simulink model "Diff_UG_2020a"  (R2020a)
settings: Solver=ode3  StartTime=0.0  StopTime=0.2  FixedStep=1e-6  RelTol=1e-3
InitFcn:
  | Ts=1/1200;
StartFcn:
  | Ts=1/1200;
undefined symbols (not defined in the file): powergui, spspowerguiLib
libraries: simulink x5, spsFourierLib x5, spsThreePhaseVIMeasurementLib x4, spsDistributedParametersLineLib x2, spsThreePhaseFaultLib x1, spsThreePhaseSeriesRLCLoadLib x1, spsThreePhaseTransformerTwoWindingsLib x1, spsThreePhaseBreakerLib x1, spsThreePhaseSourceLib x1
settings Model: Creator=AMLAN SWAIN  LastModifiedBy=mluser
settings SolverCC: ZeroCrossAlgorithm=Adaptive
settings DataIOCC: SaveFormat=StructureWithTime  ReturnWorkspaceOutputs=off
settings OptimizationCC: LifeSpan=inf
settings DebuggingCC: IgnoredZcDiagnostic=none  FcnCallInpInsideContextMsg=warning  SFExecutionAtInitializationDiag=none  ArithmeticOperatorsInVariantConditions=warning
settings HardwareCC: ProdBitPerSizeT=32  ProdBitPerPtrDiffT=32  ProdWordSize=32  ProdHWDeviceType=Specified
settings SFSimCC: CustomCodeUndefinedFunction=UseInterfaceOnly
settings CodeAppCC: StateflowObjectComments=on

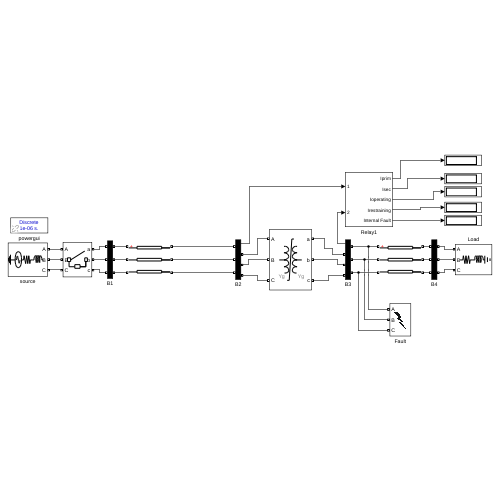
[thumbnail: Simulink's stored preview of the top-level diagram]
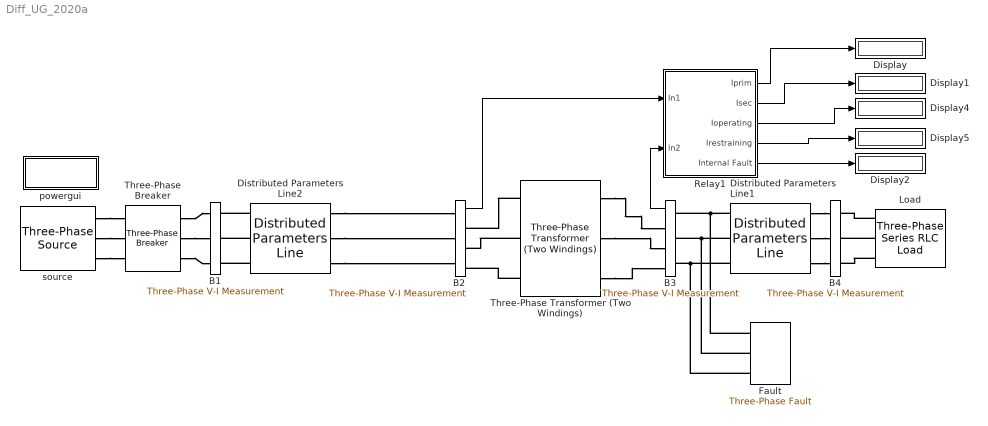
== system Diff_UG_2020a ==
  B1 : spsThreePhaseVIMeasurementLib/Three-Phase V-I Measurement  VoltageMeasurement=phase-to-phase  SetLabelV=on  LabelV=Vabc_B1  Vpu=off  VpuLL=off  CurrentMeasurement=yes  SetLabelI=on  LabelI=Iabc_B1  Ipu=off  Pbase=100e6  Vbase=500e3  OutputType=Complex  PhasorSimulation=off  PSBequivalent=0
  B2 : spsThreePhaseVIMeasurementLib/Three-Phase V-I Measurement  VoltageMeasurement=phase-to-phase  SetLabelV=on  LabelV=Vabc_B2  Vpu=off  VpuLL=off  CurrentMeasurement=yes  SetLabelI=off  LabelI=Iabc_B2  Ipu=off  Pbase=100e6  Vbase=500e3  OutputType=Complex  PhasorSimulation=off  PSBequivalent=0
  B3 : spsThreePhaseVIMeasurementLib/Three-Phase V-I Measurement  VoltageMeasurement=phase-to-phase  SetLabelV=on  LabelV=Vabc_B3  Vpu=off  VpuLL=off  CurrentMeasurement=yes  SetLabelI=off  LabelI=Iabc_B3  Ipu=off  Pbase=100e6  Vbase=500e3  OutputType=Complex  PhasorSimulation=off  PSBequivalent=0
  B4 : spsThreePhaseVIMeasurementLib/Three-Phase V-I Measurement  VoltageMeasurement=phase-to-phase  SetLabelV=on  LabelV=Vabc_B4  Vpu=off  VpuLL=off  CurrentMeasurement=yes  SetLabelI=on  LabelI=Iabc_B5  Ipu=off  Pbase=100e6  Vbase=500e3  OutputType=Complex  PhasorSimulation=off  PSBequivalent=0
  Display{,1..2,4..5} (5 alike) : Display
  Distributed Parameters Line1 : spsDistributedParametersLineLib/Distributed Parameters Line  Phases=3  Length=0.762  Frequency=60  Resistance=[0.306 0.5919]/1.6  Inductance="[0.6272  2.9855]/(2*3.14*60*1.6)"  Capacitance=[12.74e-9 7.751e-9]  x1=[-5e-06 1.09405688634751e-10 72.6531448887582 -51.7681554973917;-4e-06 1.09439141081101e-10 72.6726558603192 -51.7407622289867;-3e-06 1.09472577973709e-10 72.6921565034752 -51.7133616070655;-2e-06 1.09505999307821e-10 72.7116468154545 -51.6859536355223;-1e-06 1.09539405078689e-10 72.7311267934873 -51.6585383182524]  x2=[-5e-06 1.00008983678e-10 71.2021479909671 -51.8216475042181;-4e-06 1.00043099451765e-10 71.2216792316487 -51.7948012449423;-3e-06 1.00077201007175e-10 71.2412003501413 -51.7679476244701;-2e-06 1.00111288339383e-10 71.2607113436705 -51.741086646618;-1e-06 1.00145361443545e-10 71.2802122094634 -51.7142183152036]  x3=[-5e-06 -2.29756752635099e-12 -1.80275880533719 3.66974532044683;-4e-06 -2.29982601994123e-12 -1.80414213859099 3.66906543562833;-3e-06 -2.30208418667492e-12 -1.80552521543596 3.66838502935381;-2e-06 -2.30434202623109e-12 -1.80690803567553 3.66770410171997;-1e-06 -2.30659953828888e-12 -1.80829059911317 3.66702265282357]  x4=[-5e-06 2.59243524442771e-12 2.305788104249 -4.03237498109375;-4e-06 2.59477372905035e-12 2.30730810991507 -4.03150543293286;-3e-06 2.59711184489777e-12 2.30882778766119 -4.03063531180515;-2e-06 2.59944959163768e-12 2.31034713727139 -4.02976461783426;-1e-06 2.60178696893783e-12 2.31186615852974 -4.02889335114395]  x5=4.72092324098614e-06  V1=[9.374e-10 1.076e+04 1.076e+04;377 377 377;-1.988 0.4876 -1.083]  V2=[8.927e-10 1.062e+04 1.062e+04;377 377 377;-2.049 0.4776 -1.093]  I1=[5.305e-11 493.3 493.3;377 377 377;0.5859 3.134 1.563]  I2=[5.319e-11 560.4 560.4;377 377 377;-2.484 0.05536 -1.515]  nHarmo=1  Measurements=None  Decoupling=off  VsMag0=0  VrMag0=0  VsAngle0=0  VrAngle0=0  IsMag0=0  IrMag0=0  IsAngle0=0  IrAngle0=0
      settings: SourceProductBaseCode=PS
  Distributed Parameters Line2 : spsDistributedParametersLineLib/Distributed Parameters Line  Phases=3  Length=0.609  Frequency=60  Resistance=[0.306 0.5919]/1.6  Inductance="[0.6272  2.9855]/(2*3.14*60*1.6)"  Capacitance=[12.74e-9 7.751e-9]  x1=[-4e-06 2.33732091640896e-09 0 0;-3e-06 2.33796680931087e-09 1521.41477332637 -1004.31998129419;-2e-06 2.33861236993555e-09 1521.79328491691 -1003.74635008265;-1e-06 2.33925759819126e-09 1522.17158022669 -1003.17257621636]  x2=[-4e-06 2.33822934931859e-09 0 0;-3e-06 2.33887550786229e-09 1521.35650676479 -1004.32314155193;-2e-06 2.33952133399962e-09 1521.73501955087 -1003.74953230614;-1e-06 2.3401668276388e-09 1522.11331606446 -1003.17578040515]  x3=[-4e-06 3.406650037049e-12 0 0;-3e-06 3.40807441561528e-12 5.2142142195125 -3.32386484624876;-2e-06 3.40949830981819e-12 5.21546691648061 -3.32189889764731;-1e-06 3.41092171945535e-12 5.21671887221455 -3.31993247692994]  x4=[-4e-06 3.54043417981532e-12 0 0;-3e-06 3.54110401150702e-12 5.42755501276961 -3.70753891665244;-2e-06 3.54177333992886e-12 5.42895233629096 -3.70549251320432;-1e-06 3.54244216498573e-12 5.43034888823712 -3.70344558312308]  x5=3.77302133039443e-06  V1=[4.602e-11 2.2e+05 2.2e+05;377 377 377;2.818 0.5227 -1.048]  V2=[6.708e-11 2.2e+05 2.2e+05;377 377 377;-2.434 0.5227 -1.048]  I1=[6.93e-11 746.2 746.2;377 377 377;-1.328 0.539 -1.032]  I2=[7.511e-11 793.2 793.2;377 377 377;0.4622 0.5065 -1.064]  nHarmo=1  Measurements=None  Decoupling=off  VsMag0=0  VrMag0=0  VsAngle0=0  VrAngle0=0  IsMag0=0  IrMag0=0  IsAngle0=0  IrAngle0=0
      settings: SourceProductBaseCode=PS
  Fault : spsThreePhaseFaultLib/Three-Phase Fault  InitialStates=0  FaultA=on  FaultB=off  FaultC=off  GroundFault=on  SwitchTimes=[0.1]  External=off  SwitchStatus=NaN  FaultResistance=0.01  GroundResistance=0.01  SnubberResistance=1e6  SnubberCapacitance=inf  Measurements=None
  Load : spsThreePhaseSeriesRLCLoadLib/Three-Phase Series RLC Load  LConnTagsString=A|B|C  Configuration=Y (grounded)  NominalVoltage=4.16e3  Vabc=[1e3 1e3 1e3]*11/sqrt(3)  Vabcp=[1e3 1e3 1e3]  NominalFrequency=60  UnbalancedPower=on  ActivePower=1800e3  InductivePower=1800*0.48e3  CapacitivePower=0  Pabc=[1800e3 1800e3 1800e3]  QLabc=[872e3 872e3 872e3]  QCabc=[0 0 0 ]  Pabcp=[10e3 9e3 11e3]  QLabcp=[100 90 110]  QCabcp=[100 90 110]  Measurements=None  LoadType=constant Z
  Relay1 : Subsystem
  Three-Phase Transformer (Two Windings) : spsThreePhaseTransformerTwoWindingsLib/Three-Phase Transformer (Two Windings)  Winding1Connection=Yg  Winding2Connection=Yg  CoreType=Three single-phase transformers  SetSaturation=on  Hysteresis=off  DataFile='hysteresis'  SetInitialFlux=off  Measurements=None  UNITS=pu  NominalPower=[ 37.5e6 , 50 ]  Winding1=[220e3 , 0.01 , 0.10826]  Winding2=[11e3 , 0.01 , 0.10826 ]  Rm=500  Lm=500  L0=0.5  Saturation=[0 0;0.007 1;0.127 1.2;0.636 1.4;1.344 1.6]  InitialFluxes=[-0.0061581017798914 0.000519448171541945 0.00563865360833536]  BreakLoop=off  DiscreteSolver=Trapezoidal iterative  DataType=off  TransfoNumber=1
  Three-Phase Breaker : spsThreePhaseBreakerLib/Three-Phase Breaker  InitialState=open  SwitchA=on  SwitchB=on  SwitchC=on  SwitchTimes=[0.1]  External=off  BreakerResistance=0.01  SnubberResistance=1e6  SnubberCapacitance=inf  Measurements=None
  powergui : Subsystem  Priority=1  AncestorBlock=spspowerguiLib/powergui  DialogController=POWERSYS.PowerSysDialog  InitFcn=powergui( 'InitFcn_Callback' , gcb , 0 , [ ] );  mask(PSB option menu block){SimulationMode=Discrete, SampleTime=1e-6, frequency=60, Iterations=50, frequencyindice=0, Pbase=100e6, ErrMax=1e-4, UnitsV=kV, UnitsW=MW, buscounter=0, FunctionMessages=off, echomessages=off, EnableUseOfTLC=off, CurrentSourceSwitches=off, DisableSnubberDevices=off, DisableRonSwitches=off, DisableVfSwitches=off, DisplayEquations=off, AutomaticDiscreteSolvers=off, SolverType=Tustin/Backward Euler (TBE), Interpol=off, ExternalGateDelay=off, methode=off, Ts=100, x0status=blocks, SPID=off, SwTol=0, HookPort=off, NonlinearTolerance=1e-4, nMaxIteration=100, ContinueOnMaxIteration=off, RestoreLinks=warning, ResistiveCurrentMeasurement=off, Frange=[0:2:500], Ylog=off, Xlog=on, ShowGrid=off, save=off, variable=ZData, structure=dcneg, ZoomFFT=off, StartTime=0.1, cycles=3, DisplayStyle=1, fundamental=60, FreqAxis=off, MaxFrequency=1000, frequencyindicesteady=1, RmsSteady=1, display=off}
      mask prompts: SimulationMode "Simulation type:"; SampleTime "Sample time (s):"; frequency "Frequency (Hz):"; Iterations "Max iterations"; frequencyindice "Frequency (Hz)"; Pbase "Base power (VA)"; ErrMax "PQ tolerance (pu)"; UnitsV "Voltage units"; UnitsW "Power units"; buscounter "Load flow bus counter"; FunctionMessages "Disable Specialized Power Systems warnings"; echomessages "Display Specialized Power Systems compilation messages"; EnableUseOfTLC "Use TLC file when in Accelerator Simulation Mode and for code generation"; CurrentSourceSwitches "Disable ideal switching"; DisableSnubberDevices "Disable snubbers in switching devices"; DisableRonSwitches "Disable Ron resistances in switching devices"; DisableVfSwitches "Disable forward voltages in switching devices"; DisplayEquations "Display circuit differential equations"; AutomaticDiscreteSolvers "Automatically handle Discrete solver and Advanced tab solver settings of blocks"; SolverType "Discrete solver"; Interpol "Interpolate switching events"; ExternalGateDelay "Use time-stamped gate signals"; methode "Store switching topologies"; Ts "Buffer size (MBytes):"; x0status "Start simulation with initial electrical states from:"; SPID "Use ideal switching devices"; SwTol "Switch tolerance"; HookPort "Allow multiple powergui blocks"; NonlinearTolerance "Solver tolerance"; nMaxIteration "Maximum number of iterations"; ContinueOnMaxIteration "Continue Simulation if maximum number of iterations is reached"; RestoreLinks "Restore disabled links of Simscape Power Systems ST blocks:"; ResistiveCurrentMeasurement "Use non ideal current measurement blocks (1e-4Ohm internal resistance)"; Frange "Frequency Range"; Ylog "Log impedance"; Xlog "log Frequency"; ShowGrid "grid"; save "Save Data To Workspace"; variable "Variable Name"; structure "Structure Name (PSBFFTSCOPE)"; ZoomFFT "ZoomFFT (PSBFFTSCOPE)"; StartTime "Start Time (PSBFFTSCOPE)"; cycles "Cycles (PSBFFTSCOPE)"; DisplayStyle "Display style (PSBFFTSCOPE)"; fundamental "Fundamental (PSBFFTSCOPE)"; FreqAxis "Frequency Axis (PSBFFTSCOPE)"; MaxFrequency "Max Frequency (PSBFFTSCOPE)"; frequencyindicesteady "Frequency indice (STEADYSTATE)"; RmsSteady "RMS display (STEADYSTATE)"; display "Display Results"
      mask help: Set simulation type, simulation parameters, and preferences.
      mask init:
      | dispMessage = powergui('MaskInitialization',gcb,SimulationMode,SampleTime);
      settings: PreSaveFcn=powergui( 'PreSaveFcn_Callback' , gcb , [ ] , [ ] );  OpenFcn=sps_rtmsupport('OpenFcn',gcbh)
      mask Help: helpview(psbhelp)
      mask TypeOptions SimulationMode: Continuous | Discrete | Phasor | Discrete phasor
      mask Callback SimulationMode: powergui('SimulationType',[],[],gcb);
      mask TypeOptions UnitsV: V | kV
      mask TypeOptions UnitsW: W | kW | MW
      mask Callback CurrentSourceSwitches: powergui('SimulationType',[],[],gcb);
      mask Callback AutomaticDiscreteSolvers: powergui('SimulationType',[],[],gcb);
      mask TypeOptions SolverType: Tustin/Backward Euler (TBE) | Tustin | Backward Euler
      mask Callback SolverType: powergui('SimulationType',[],[],gcb);
      mask Callback Interpol: powergui('SimulationType',[],[],gcb);
      mask Callback ExternalGateDelay: powergui('SimulationType',[],[],gcb);
      mask Callback methode: powergui('SimulationType',[],[],gcb);
      mask TypeOptions x0status: blocks | steady | zero
      mask TypeOptions RestoreLinks: yes | warning | no
      mask Callback display: sps_rtmsupport('parametereditingmodes',gcbh) % Will be executed last in parameter callbacks to ensure mask enable consistency
      mask DialogControl SolverTab Prompt: Solver
      mask DialogControl AutoSolverNote Prompt: The Simulation type parameter is governed by Simulink. To access the Powergui solver settings, unselect auto (Automatic solver selection) solver in the Simulink solver options.
      mask DialogControl Container15 Prompt: Tools
      mask DialogControl StateAnalyzer Prompt: Measurements and States Analyzer
      mask DialogControl StateAnalyzer Callback: powerStates(bdroot(gcb))
      mask DialogControl RLCLineParameters Prompt: Power Line Parameters
      mask DialogControl RLCLineParameters Callback:
      | close_system(gcb)
      | powerLineParameters
      mask DialogControl DecouplingLines Prompt: Specify Decoupling Lines
      mask DialogControl DecouplingLines Tooltip: Click to replace selected Distributed Parameters Line blocks with Decoupling Line blocks
      mask DialogControl DecouplingLines Callback:
      | close_system(gcb);
      | DecouplingLineReplace(gcs)
      mask DialogControl LoadFlow Prompt: Load Flow Analyzer
      mask DialogControl LoadFlow Callback:
      | close_system(gcb)
      | powerLoadFlow
      mask DialogControl Container11 Prompt: Load Flow Parameters
      mask DialogControl MachineInitialization Prompt: Machine Initialization
      mask DialogControl MachineInitialization Callback:
      | close_system(gcb)
      | powericon('machineInitTool',bdroot(gcb),gcb)
      mask DialogControl ImpedanceMeasurement Prompt: Impedance Measurement
      mask DialogControl ImpedanceMeasurement Callback:
      | close_system(gcb);
      | powerImpedance(bdroot(gcs));
      mask DialogControl FFTAnalysis Prompt: FFT Analysis
      mask DialogControl FFTAnalysis Callback:
      | close_system(gcb)
      | power_fftscope(bdroot(gcb),gcb)
      mask DialogControl LinearSystemAnalyzer Prompt: Use Linear System Analyzer
      mask DialogControl LinearSystemAnalyzer Callback:
      | close_system(gcb)
      | power_ltiview(bdroot(gcb))
      mask DialogControl HysteresisDesign Prompt: Hysteresis Design
      mask DialogControl HysteresisDesign Callback:
      | close_system(gcb)
      | powerHysteresis('hysteresis.mat')
      mask DialogControl Control14 Prompt: Customize SPS blocks
      mask DialogControl Control14 Callback:
      | close_system(gcb);
      | power_customize;
      mask DialogControl GenerateReprot Prompt: Generate Report
      mask DialogControl GenerateReprot Callback:
      | close_system(gcb)
      | power_report(bdroot(gcb))
      mask DialogControl ParameterTabVar012 Prompt: Preferences
      mask DialogControl Solver Prompt: Solver
      mask DialogControl SolverDetails Prompt: Solver details for nonlinear elements
      mask Display: color('blue'),disp(dispMessage)
  source : spsThreePhaseSourceLib/Three-Phase Source  InternalConnection=Yg  VoltagePhases=off  Voltage=220e3  PhaseAngle=0  Voltage_phases=[220e3 220e3 220e3]/sqrt(3)  PhaseAngles_phases=[0]  Frequency=60  NonIdealSource=on  SpecifyImpedance=on  Resistance=0.8929  Inductance=0.025  ShortCircuitLevel=60000e6  BaseVoltage=220e3  XRratio=7  BusType=swing  Pref=10e3  Qref=0  Prefabc=[10e3, 10e3, 10e3]  Qrefabc=[0, 0, 0]  Qmin=-inf  Qmax=inf
  wires:
  B2/1 -> Relay1/1(In1)
  B3/1 -> Relay1/2(In2)
  Relay1/1(Iprim) -> Display/1
  Relay1/2(Isec) -> Display1/1
  Relay1/5(Internal Fault) -> Display2/1
  Relay1/3(Ioperating) -> Display4/1
  Relay1/4(Irestraining) -> Display5/1
  connections:
  Load/LConn1 -- B4/LConn1
  Load/LConn2 -- B4/LConn2
  Load/LConn3 -- B4/LConn3
  Three-Phase Transformer (Two Windings)/RConn3 -- B3/RConn3
  Distributed Parameters Line1/LConn1 -- Fault/LConn1 -- B3/LConn1
  Distributed Parameters Line1/LConn2 -- Fault/LConn2 -- B3/LConn2
  Distributed Parameters Line1/LConn3 -- Fault/LConn3 -- B3/LConn3
  Distributed Parameters Line1/RConn1 -- B4/RConn1
  Distributed Parameters Line1/RConn2 -- B4/RConn2
  Distributed Parameters Line1/RConn3 -- B4/RConn3
  Distributed Parameters Line2/RConn1 -- B2/LConn1
  Distributed Parameters Line2/RConn2 -- B2/LConn2
  Distributed Parameters Line2/RConn3 -- B2/LConn3
  Distributed Parameters Line2/LConn1 -- B1/RConn1
  Distributed Parameters Line2/LConn2 -- B1/RConn2
  Distributed Parameters Line2/LConn3 -- B1/RConn3
  Three-Phase Transformer (Two Windings)/LConn2 -- B2/RConn2
  Three-Phase Transformer (Two Windings)/LConn1 -- B2/RConn1
  Three-Phase Transformer (Two Windings)/LConn3 -- B2/RConn3
  source/RConn1 -- Three-Phase Breaker/LConn1
  source/RConn2 -- Three-Phase Breaker/LConn2
  source/RConn3 -- Three-Phase Breaker/LConn3
  Three-Phase Breaker/RConn2 -- B1/LConn2
  Three-Phase Breaker/RConn1 -- B1/LConn1
  Three-Phase Breaker/RConn3 -- B1/LConn3
  Three-Phase Transformer (Two Windings)/RConn2 -- B3/RConn2
  Three-Phase Transformer (Two Windings)/RConn1 -- B3/RConn1

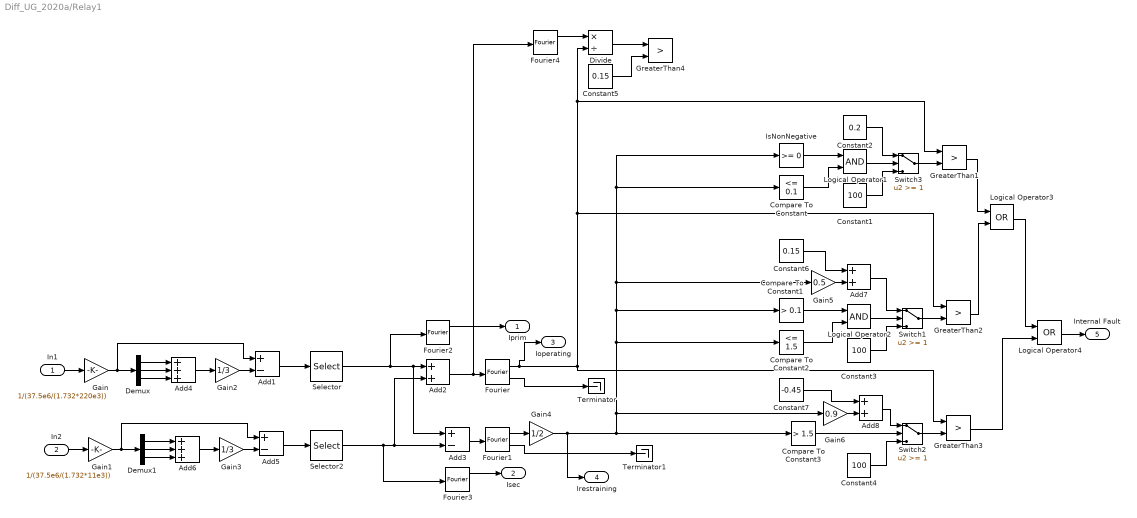
== system Diff_UG_2020a/Relay1 ==
  In1 : Inport
  In2 : Inport  Port=2
  Add1 : Sum  Inputs=+-
  Add2 : Sum
  Add3 : Sum  Inputs=+-
  Add4 : Sum  Inputs=+++
  Add5 : Sum  Inputs=+-
  Add6 : Sum  Inputs=+++
  Add7 : Sum
  Add8 : Sum
  Compare To Constant : simulink/Logic and Bit Operations/Compare To Constant  relop=<=  const=0.1  OutDataTypeStr=boolean
  Compare To Constant1 : simulink/Logic and Bit Operations/Compare To Constant  relop=>  const=0.1  OutDataTypeStr=boolean
  Compare To Constant2 : simulink/Logic and Bit Operations/Compare To Constant  relop=<=  const=1.5  OutDataTypeStr=boolean
  Compare To Constant3 : simulink/Logic and Bit Operations/Compare To Constant  relop=>  const=1.5  OutDataTypeStr=boolean
  Constant1 : Constant  Value=100
  Constant2 : Constant  Value=0.2
  Constant3 : Constant  Value=100
  Constant4 : Constant  Value=100
  Constant5 : Constant  Value=0.15
  Constant6 : Constant  Value=0.15
  Constant7 : Constant  Value=-0.45
  Demux : Demux  Outputs=3
  Demux1 : Demux  Outputs=3
  Divide : Product  Inputs=*/
  Fourier{,1..3} (4 alike) : spsFourierLib/Fourier  Freq=60  n=1  InInit=[0, 0]  Ts=0
      settings: SourceProductBaseCode=PS
  Fourier4 : spsFourierLib/Fourier  Freq=60  n=2  InInit=[0, 0]  Ts=0
      settings: SourceProductBaseCode=PS
  Gain : Gain  Gain=1/(37.5e6/(1.732*220e3))
  Gain1 : Gain  Gain=1/(37.5e6/(1.732*11e3))
  Gain2 : Gain  Gain=1/3
  Gain3 : Gain  Gain=1/3
  Gain4 : Gain  Gain=1/2
  Gain5 : Gain  Gain=0.5
  Gain6 : Gain  Gain=0.9
  GreaterThan{1..4} (4 alike) : RelationalOperator  Operator=>  OutDataTypeStr=boolean  RndMeth=Nearest
  IsNonNegative : simulink/Logic and Bit Operations/Compare To Zero  relop=>=  OutDataTypeStr=boolean
  Logical Operator1 : Logic  AllPortsSameDT=off  OutDataTypeStr=boolean
  Logical Operator2 : Logic  AllPortsSameDT=off  OutDataTypeStr=boolean
  Logical Operator3 : Logic  Operator=OR  AllPortsSameDT=off  OutDataTypeStr=boolean
  Logical Operator4 : Logic  Operator=OR  AllPortsSameDT=off  OutDataTypeStr=boolean
  Selector : Selector  InputPortWidth=3  IndexOptions=Index vector (dialog)  Indices=[1]  OutputSizes=1
  Selector2 : Selector  InputPortWidth=3  IndexOptions=Index vector (dialog)  Indices=[1]  OutputSizes=1
  Switch1 : Switch  Threshold=1
  Switch2 : Switch  Threshold=1
  Switch3 : Switch  Threshold=1
  Terminator : Terminator
  Terminator1 : Terminator
  Iprim : Outport
  Isec : Outport  Port=2
  Ioperating : Outport  Port=3
  Irestraining : Outport  Port=4
  Internal Fault : Outport  Port=5
  wires:
  Add2/1 -> Fourier4/1, Fourier/1
  In2/1 -> Gain1/1
  In1/1 -> Gain/1
  Fourier/2 -> Terminator/1
  Add3/1 -> Fourier1/1
  Fourier1/1 -> Gain4/1
  Fourier1/2 -> Terminator1/1
  Demux/1 -> Add4/1
  Demux/2 -> Add4/2
  Demux/3 -> Add4/3
  Add4/1 -> Gain2/1
  Gain2/1 -> Add1/2
  Gain/1 -> Add1/1, Demux/1
  Demux1/2 -> Add6/2
  Add6/1 -> Gain3/1
  Gain3/1 -> Add5/2
  Demux1/1 -> Add6/1
  Demux1/3 -> Add6/3
  Gain1/1 -> Add5/1, Demux1/1
  Constant2/1 -> Switch3/1
  IsNonNegative/1 -> Logical Operator1/1
  Compare To Constant/1 -> Logical Operator1/2
  Logical Operator1/1 -> Switch3/2
  Constant1/1 -> Switch3/3
  GreaterThan1/1 -> Logical Operator3/1
  Switch3/1 -> GreaterThan1/2
  Compare To Constant2/1 -> Logical Operator2/2
  Compare To Constant1/1 -> Logical Operator2/1
  Logical Operator2/1 -> Switch1/2
  Switch1/1 -> GreaterThan2/2
  Constant3/1 -> Switch1/3
  Switch2/1 -> GreaterThan3/2
  Compare To Constant3/1 -> Switch2/2
  Constant4/1 -> Switch2/3
  GreaterThan3/1 -> Logical Operator4/2
  Fourier/1 -> Ioperating/1, GreaterThan3/1, GreaterThan2/1, Divide/2, GreaterThan1/1
  Gain4/1 -> Irestraining/1, Compare To Constant3/1, Compare To Constant2/1, Compare To Constant1/1, Gain5/1, Compare To Constant/1, IsNonNegative/1, Gain6/1
  Fourier2/1 -> Iprim/1
  Fourier3/1 -> Isec/1
  GreaterThan2/1 -> Logical Operator3/2
  Logical Operator3/1 -> Logical Operator4/1
  Logical Operator4/1 -> Internal Fault/1
  Add1/1 -> Selector/1
  Selector/1 -> Fourier2/1, Add3/1, Add2/1
  Add5/1 -> Selector2/1
  Selector2/1 -> Fourier3/1, Add3/2, Add2/2
  Fourier4/1 -> Divide/1
  Divide/1 -> GreaterThan4/1
  Constant5/1 -> GreaterThan4/2
  Gain5/1 -> Add7/2
  Add7/1 -> Switch1/1
  Constant6/1 -> Add7/1
  Gain6/1 -> Add8/2
  Add8/1 -> Switch2/1
  Constant7/1 -> Add8/1

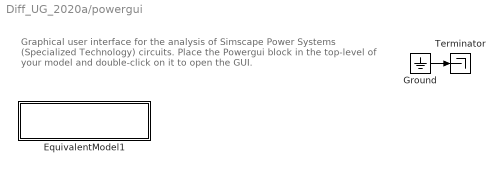
== system Diff_UG_2020a/powergui ==
  note: Graphical user interface for the analysis of
      | Simscape Power Systems (Specialized Technology) circuits.
      | Place the Powergui block in the top-level of your model and double-click
      | on it to open the GUI.
  EquivalentModel1 : Subsystem
      mask init:
      | S  = GetDataForEquivalentModel('Discrete',gcbh);
      mask Display:
      | color('red')
      | disp('EQUIVALENT CIRCUIT\nDiscrete')
  Ground : Ground
  Terminator : Terminator
  wires:
  Ground/1 -> Terminator/1

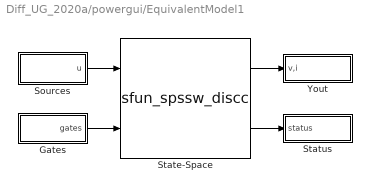
== system Diff_UG_2020a/powergui/EquivalentModel1 ==
  Gates : Subsystem
  Sources : Subsystem
  State-Space : S-Function  FunctionName=sfun_spssw_discc  Parameters=S.Ts,S.A, S.B, S.C, S.D, S.x0, S.EnableUseOfTLC,S.SwitchResistance ,S.SwitchType, S.SwitchGateInitialValue, S.OutputsToResetToZero, S.TBEON,S.SaveMatrices,S.BufferSize  SFunctionDeploymentMode=off  EnableBusSupport=off
  Status : Subsystem
  Yout : Subsystem
  wires:
  Gates/1(gates) -> State-Space/2
  Sources/1(u) -> State-Space/1
  State-Space/2 -> Status/1(status)
  State-Space/1 -> Yout/1(v,i)

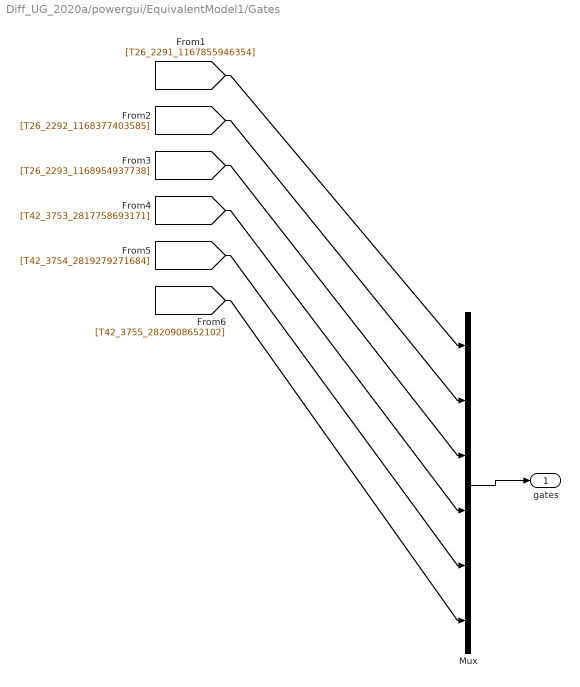
== system Diff_UG_2020a/powergui/EquivalentModel1/Gates ==
  Mux : Mux  Inputs=[1 1 1 1 1 1]
  gates : Outport  VectorParamsAs1DForOutWhenUnconnected=off
  wires:
  Mux/1 -> gates/1
  [T26_2291_1167855946354] -> Mux/1
  [T26_2292_1168377403585] -> Mux/2
  [T26_2293_1168954937738] -> Mux/3
  [T42_3753_2817758693171] -> Mux/4
  [T42_3754_2819279271684] -> Mux/5
  [T42_3755_2820908652102] -> Mux/6

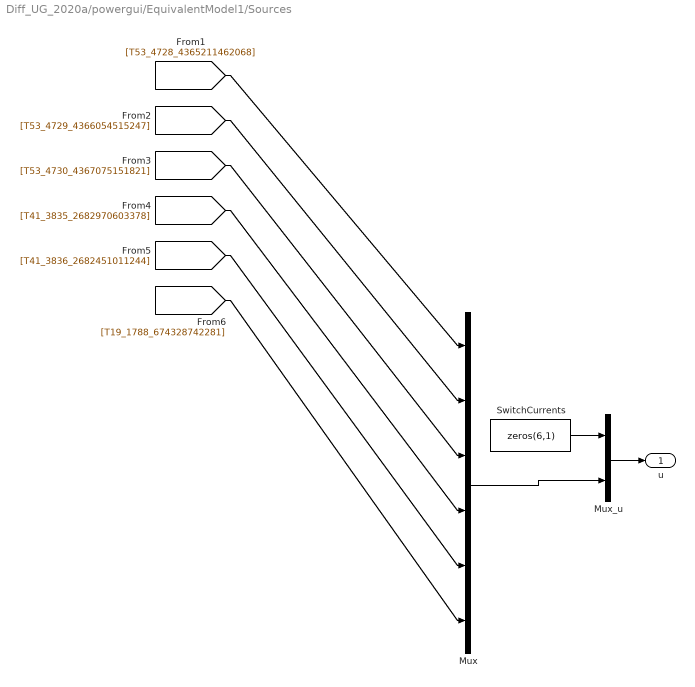
== system Diff_UG_2020a/powergui/EquivalentModel1/Sources ==
  Mux : Mux  Inputs=[1 1 1 6 6 3]
  Mux_u : Mux  Inputs=[6 18]
  SwitchCurrents : Constant  Value=zeros(6,1)
  u : Outport  VectorParamsAs1DForOutWhenUnconnected=off
  wires:
  Mux_u/1 -> u/1
  SwitchCurrents/1 -> Mux_u/1
  Mux/1 -> Mux_u/2
  [T53_4728_4365211462068] -> Mux/1
  [T53_4729_4366054515247] -> Mux/2
  [T53_4730_4367075151821] -> Mux/3
  [T41_3835_2682970603378] -> Mux/4
  [T41_3836_2682451011244] -> Mux/5
  [T19_1788_674328742281] -> Mux/6

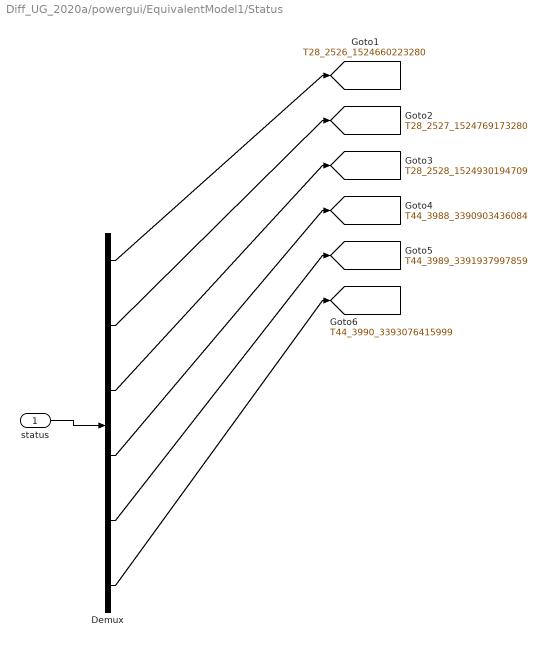
== system Diff_UG_2020a/powergui/EquivalentModel1/Status ==
  status : Inport
  Demux : Demux  Outputs=[1 1 1 1 1 1]
  tag scope: T28_2526_1524660223280=global, T28_2527_1524769173280=global, T28_2528_1524930194709=global, T44_3988_3390903436084=global, T44_3989_3391937997859=global, T44_3990_3393076415999=global
  wires:
  status/1 -> Demux/1
  Demux/1 -> [T28_2526_1524660223280]
  Demux/2 -> [T28_2527_1524769173280]
  Demux/3 -> [T28_2528_1524930194709]
  Demux/4 -> [T44_3988_3390903436084]
  Demux/5 -> [T44_3989_3391937997859]
  Demux/6 -> [T44_3990_3393076415999]

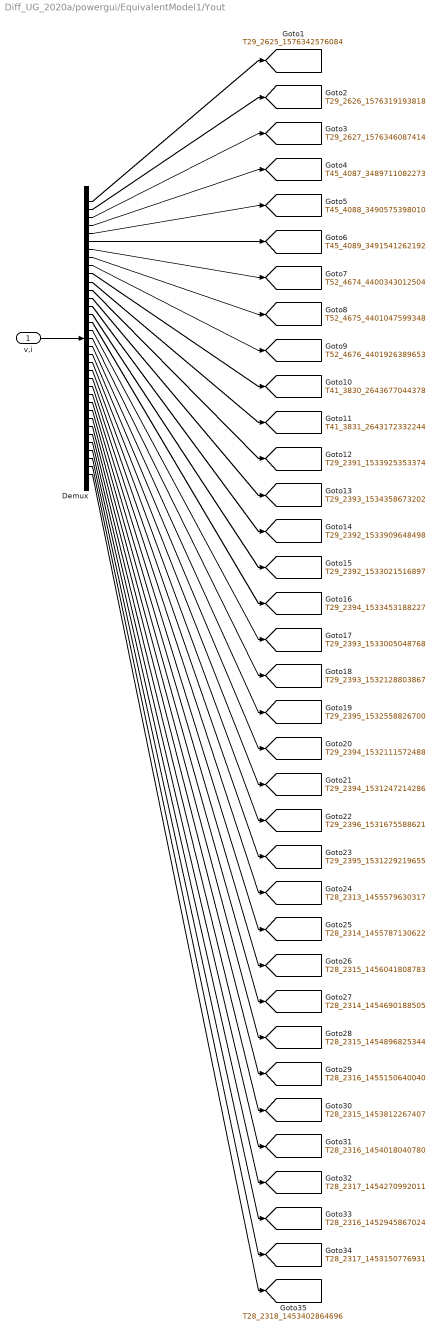
== system Diff_UG_2020a/powergui/EquivalentModel1/Yout ==
  v,i : Inport
  Demux : Demux  Outputs=[1 1 1 1 1 1 1 1 1 6 6 1 1 1 1 1 1 1 1 1 1 1 1 1 1 1 1 1 1 1 1 1 1 1 1]
  tag scope: T28_2313_1455579630317=global, T28_2314_1454690188505=global, T28_2314_1455787130622=global, T28_2315_1453812267407=global, T28_2315_1454896825344=global, T28_2315_1456041808783=global, T28_2316_1452945867024=global, T28_2316_1454018040780=global, T28_2316_1455150640040=global, T28_2317_1453150776931=global, T28_2317_1454270992011=global, T28_2318_1453402864696=global, T29_2391_1533925353374=global, T29_2392_1533021516897=global, T29_2392_1533909648498=global, T29_2393_1532128803867=global, T29_2393_1533005048768=global, T29_2393_1534358673202=global, T29_2394_1531247214286=global, T29_2394_1532111572488=global, T29_2394_1533453188227=global, T29_2395_1531229219655=global, T29_2395_1532558826700=global, T29_2396_1531675588621=global, T29_2625_1576342576084=global, T29_2626_1576319193818=global, T29_2627_1576346087414=global, T41_3830_2643677044378=global, T41_3831_2643172332244=global, T45_4087_3489711082273=global, T45_4088_3490575398010=global, T45_4089_3491541262192=global, T52_4674_4400343012504=global, T52_4675_4401047599348=global, T52_4676_4401926389653=global
  wires:
  v,i/1 -> Demux/1
  Demux/1 -> [T29_2625_1576342576084]
  Demux/2 -> [T29_2626_1576319193818]
  Demux/3 -> [T29_2627_1576346087414]
  Demux/4 -> [T45_4087_3489711082273]
  Demux/5 -> [T45_4088_3490575398010]
  Demux/6 -> [T45_4089_3491541262192]
  Demux/7 -> [T52_4674_4400343012504]
  Demux/8 -> [T52_4675_4401047599348]
  Demux/9 -> [T52_4676_4401926389653]
  Demux/10 -> [T41_3830_2643677044378]
  Demux/11 -> [T41_3831_2643172332244]
  Demux/12 -> [T29_2391_1533925353374]
  Demux/13 -> [T29_2393_1534358673202]
  Demux/14 -> [T29_2392_1533909648498]
  Demux/15 -> [T29_2392_1533021516897]
  Demux/16 -> [T29_2394_1533453188227]
  Demux/17 -> [T29_2393_1533005048768]
  Demux/18 -> [T29_2393_1532128803867]
  Demux/19 -> [T29_2395_1532558826700]
  Demux/20 -> [T29_2394_1532111572488]
  Demux/21 -> [T29_2394_1531247214286]
  Demux/22 -> [T29_2396_1531675588621]
  Demux/23 -> [T29_2395_1531229219655]
  Demux/24 -> [T28_2313_1455579630317]
  Demux/25 -> [T28_2314_1455787130622]
  Demux/26 -> [T28_2315_1456041808783]
  Demux/27 -> [T28_2314_1454690188505]
  Demux/28 -> [T28_2315_1454896825344]
  Demux/29 -> [T28_2316_1455150640040]
  Demux/30 -> [T28_2315_1453812267407]
  Demux/31 -> [T28_2316_1454018040780]
  Demux/32 -> [T28_2317_1454270992011]
  Demux/33 -> [T28_2316_1452945867024]
  Demux/34 -> [T28_2317_1453150776931]
  Demux/35 -> [T28_2318_1453402864696]
